simulink model "New_xiezuo_joint_controller_verification_H25_motor"  (R2020b)
settings: Solver=FixedStepAuto  StartTime=0.0  StopTime=25  FixedStep=0.00001  RelTol=1e-4
InitFcn:
  | Ts = 10e-6;
  | 
  | R = 0.958;
  | Ld = 5.25e-3;
  | Lq = 12e-3;
  | Pn = 4;
  | flux = 0.1827;
model workspace (MAT data in the model file):
  Flux_Linkage = 0.027213034
  Torque_Constant = 0.2885
  Voltage_Constant = 30.23
libraries: pid_lib x1
settings Model: Creator=SUN  LastModifiedBy=baikp
settings SolverCC: ZeroCrossControl=DisableAll
settings DataIOCC: LimitDataPoints=on  SaveFormat=Array  SignalLoggingSaveFormat=ModelDataLogs  ReturnWorkspaceOutputs=off
settings OptimizationCC: ExpressionDepthLimit=2147483647  InitFltsAndDblsToZero=on  LifeSpan=inf
settings DebuggingCC: UnderspecifiedInitializationDetection=Classic  MergeDetectMultiDrivingBlocksExec=none  SolverPrmCheckMsg=warning  FcnCallInpInsideContextMsg=warning  StateNameClashWarn=warning  SFUnexpectedBacktrackingDiag=warning  SFNoUnconditionalDefaultTransitionDiag=warning  SFExecutionAtInitializationDiag=none  ArithmeticOperatorsInVariantConditions=warning
settings HardwareCC: ProdBitPerPointer=32  ProdBitPerSizeT=32  ProdBitPerPtrDiffT=32  ProdLargestAtomicFloat=None  ProdIntDivRoundTo=Undefined  ProdEndianess=Unspecified  ProdWordSize=32  ProdHWDeviceType=32-bit Generic
settings ModelReferenceCC: PropagateSignalLabelsOutOfModel=off
settings SFSimCC: SimUseLocalCustomCode=off  CustomCodeUndefinedFunction=UseInterfaceOnly
settings RTWCC: RTWUseLocalCustomCode=off
settings CodeAppCC: StateflowObjectComments=on
settings GRTTargetCC: TargetLangStandard=C89/C90 (ANSI)  CombineOutputUpdateFcns=off  GRTInterface=on
settings ConfigComp: CovMetricSettings=dw  CovSaveCumulativeToWorkspaceVar=on  CovSaveSingleToWorkspaceVar=on  CovExternalEMLEnable=off  CovSFcnEnable=off
settings SimscapeCC: SimscapeNormalizeSystem=off

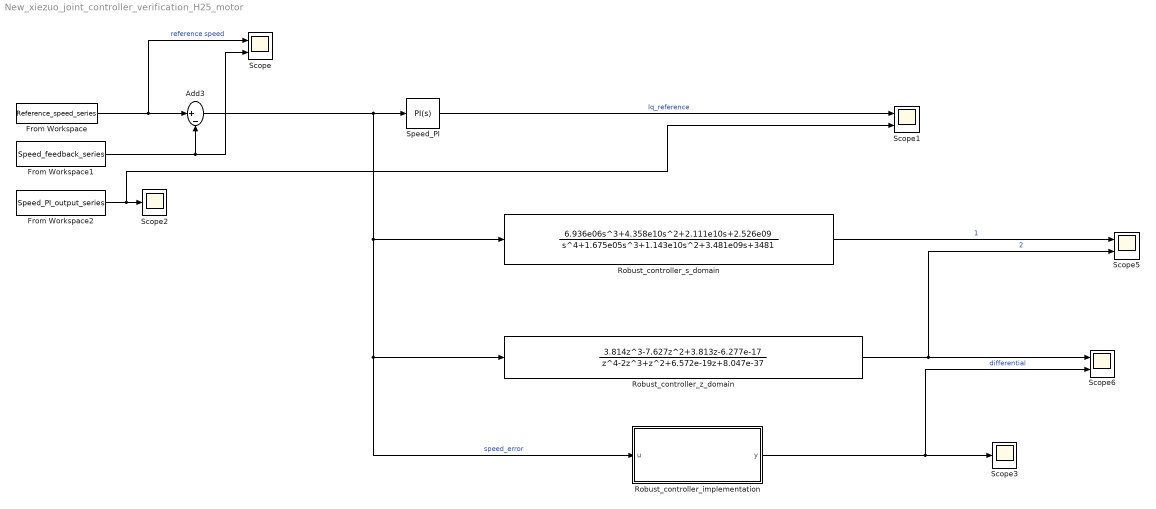
== system New_xiezuo_joint_controller_verification_H25_motor ==
  Add3 : Sum  Inputs=|+-
  From Workspace : FromWorkspace  VariableName=Reference_speed_series  SampleTime=-1
  From Workspace1 : FromWorkspace  VariableName=Speed_feedback_series  SampleTime=-1
  From Workspace2 : FromWorkspace  VariableName=Speed_PI_output_series  SampleTime=-1
  Robust_controller_implementation : Subsystem
  Robust_controller_s_domain : TransferFcn  Numerator=[6.936e06 4.358e10 2.111e10 2.526e09]  Denominator=[1 1.675e05 1.143e10 3.481e09 3481]
  Robust_controller_z_domain : DiscreteTransferFcn  Numerator=[3.814 -7.627 3.813 -6.277e-17]  Denominator=[1 -2 1 6.572e-19 8.047e-37]  SampleTime=0.0005
  Scope{,1,5..6} (4 alike) : Scope  NumInputPorts=2
  Scope2 : Scope
  Scope3 : Scope
  Speed_PI : pid_lib/PID Controller  Controller=PI  Form=Parallel  TimeDomain=Continuous-time  UseExternalTs=off  SampleTime=0.0005  IntegratorMethod=Forward Euler  FilterMethod=Forward Euler  ControllerParametersSource=internal  P=4.5  I=180.6  D=0  UseFilter=on  N=100  TunerSelectOption=Transfer Function Based (PID Tuner App)  InitialConditionSource=internal  InitialConditionForIntegrator=0  InitialConditionForFilter=0  DifferentiatorICPrevScaledInput=0  ExternalReset=none  TrackingMode=off  Kt=1  LimitOutput=off  SatLimitsSource=internal  UpperSaturationLimit=inf  LowerSaturationLimit=-inf  LinearizeAsGain=on  AntiWindupMode=none  Kb=1  POutMin=[]  POutMax=[]  IOutMin=[]  IOutMax=[]  DOutMin=[]  DOutMax=[]  NOutMin=[]  NOutMax=[]  SumOutMin=[]  SumOutMax=[]  SaturationOutMin=[]  SaturationOutMax=[]  PParamMin=[]  PParamMax=[]  IParamMin=[]  IParamMax=[]  DParamMin=[]  DParamMax=[]  NParamMin=[]  NParamMax=[]  KbParamMin=[]  KbParamMax=[]  KtParamMin=[]  KtParamMax=[]  KbOutMin=[]  KbOutMax=[]  KtOutMin=[]  KtOutMax=[]  IntegratorOutMin=[]  IntegratorOutMax=[]  FilterOutMin=[]  FilterOutMax=[]  SumI1OutMin=[]  SumI1OutMax=[]  SumI2OutMin=[]  SumI2OutMax=[]  SumI3OutMin=[]  SumI3OutMax=[]  SumI4OutMin=[]  SumI4OutMax=[]  SumDOutMin=[]  SumDOutMax=[]  DifferentiatorOutMin=[]  DifferentiatorOutMax=[]  FilterDiffOutCoefMin=[]  FilterDiffOutCoefMax=[]  ReciprocalOutMin=[]  ReciprocalOutMax=[]  SumDenOutMin=[]  SumDenOutMax=[]  SumNumOutMin=[]  SumNumOutMax=[]  DivideOutMin=[]  DivideOutMax=[]  UdiffTsProdOutMin=[]  UdiffTsProdOutMax=[]  NTsProdOutMin=[]  NTsProdOutMax=[]  UintegralTsProdOutMin=[]  UintegralTsProdOutMax=[]  UngainTsProdOutMin=[]  UngainTsProdOutMax=[]  IntegratorContinuousStateAttributes=''  IntegratorStateMustResolveToSignalObject=off  IntegratorRTWStateStorageClass=Auto  FilterContinuousStateAttributes=''  FilterStateMustResolveToSignalObject=off  FilterRTWStateStorageClass=Auto  ParallelPVariant=InternalParameters  IdealPVariant=Disabled  IVariant=InternalParameters  DVariant=Disabled  IntegratorVariant=Continuous  SatVariant=Disabled  AWVariant=Passthrough  PCopyVariant=Disabled  TRVariant=Disabled  FdbkBlocksVariant=Forward  IdealPFdbkVariant=Disabled  SatFdbkVariant=Disabled  DerivativeFilterVariant=Disabled  NVariant=Disabled  NCopyVariant=Disabled_SignalSpec  FilterICVariant=Disabled  IntegratorICVariant=InternalICs  ExternalResetVariant=Disabled  TRSumVariant=Passthrough  SumFdbkVariant=Disabled  SumVariant=Sum_PI  TsampFilterVariant=InternalTs  TsampNgainVariant=Passthrough  TsampIntegralVariant=Passthrough  ExternalSaturationOutDataTypeStr=Inherit: Same as second input
  wires:
  Add3/1 -> Robust_controller_implementation/1(u), Robust_controller_z_domain/1, Robust_controller_s_domain/1, Speed_PI/1  "speed_error"
  Speed_PI/1 -> Scope1/1  "Iq_reference"
  From Workspace/1 -> Scope/1, Add3/1  "reference speed"
  From Workspace1/1 -> Scope/2, Add3/2
  From Workspace2/1 -> Scope1/2, Scope2/1
  Robust_controller_s_domain/1 -> Scope5/1  "1"
  Robust_controller_z_domain/1 -> Scope5/2, Scope6/1  "2"
  Robust_controller_implementation/1(y) -> Scope6/2, Scope3/1  "differential"

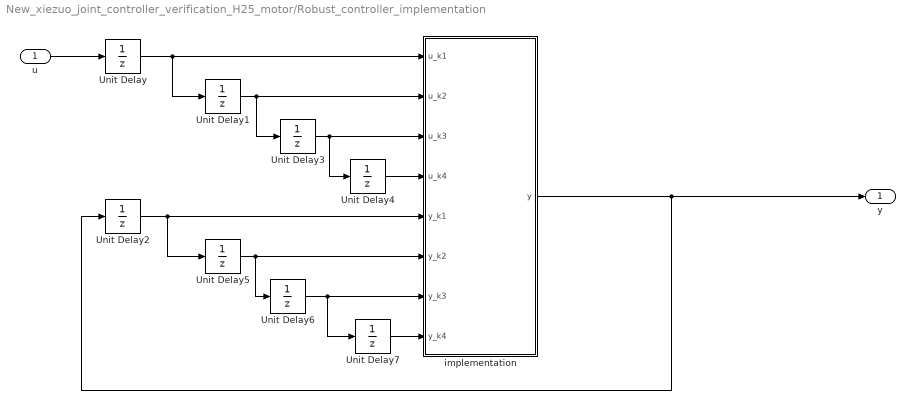
== system New_xiezuo_joint_controller_verification_H25_motor/Robust_controller_implementation ==
  u : Inport
  Unit Delay{,1..7} (8 alike) : UnitDelay  SampleTime=0.0005  HasFrameUpgradeWarning=on
  implementation : MATLAB Function  TreatAsAtomicUnit=on
  y : Outport
  wires:
  implementation/1(y) -> Unit Delay2/1, y/1
  u/1 -> Unit Delay/1
  Unit Delay/1 -> Unit Delay1/1, implementation/1(u_k1)
  Unit Delay1/1 -> Unit Delay3/1, implementation/2(u_k2)
  Unit Delay3/1 -> Unit Delay4/1, implementation/3(u_k3)
  Unit Delay4/1 -> implementation/4(u_k4)
  Unit Delay2/1 -> Unit Delay5/1, implementation/5(y_k1)
  Unit Delay5/1 -> Unit Delay6/1, implementation/6(y_k2)
  Unit Delay6/1 -> Unit Delay7/1, implementation/7(y_k3)
  Unit Delay7/1 -> implementation/8(y_k4)

== matlab function New_xiezuo_joint_controller_verification_H25_motor/Robust_controller_implementation/implementation ==
  data: y output; u_k1 input; u_k2 input; u_k3 input; u_k4 input; y_k1 input; y_k2 input; y_k3 input; y_k4 input
function y = fcn(u_k1,u_k2,u_k3,u_k4,y_k1,y_k2,y_k3,y_k4)

y = 2*y_k1 - y_k2 - 6.572e-19*y_k3 - 8.047e-37*y_k4 + 3.814*u_k1 - 7.627*u_k2 + 3.813*u_k3 - 6.277e-17*u_k4;
